simulink model "Model_Proportional"  (R2014b)
settings: Solver=ode45  StartTime=0.0  StopTime=30  RelTol=1e-6
values from neighbouring files (symbols this model uses):
  Kp = Ki    [Main.m]    (also in Q1_UsingTF.m = Kpv(i); Q2_UsingTF.m = 0; Q3_UsingTF.m; RunSimModel.m = 0)
settings Model: Creator=Eduardo  LastModifiedBy=Eduardo

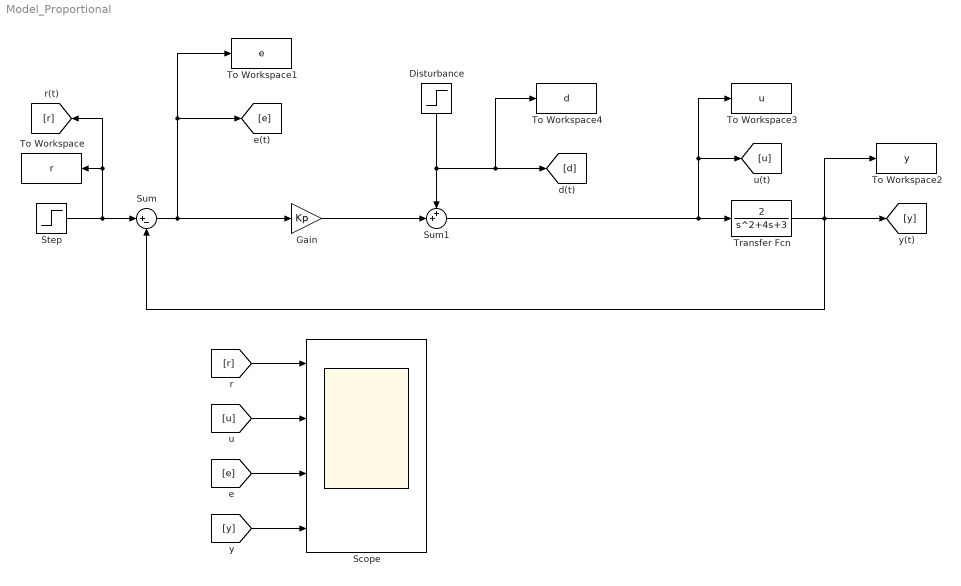
== system Model_Proportional ==
  Disturbance : Step  Time=0  After=0  SampleTime=0
  Gain : Gain  Gain=Kp
  Scope : Scope  NumInputPorts=4
      settings: YMin=-5~-5~-5~-5  YMax=5~5~5~5
  Step : Step  SampleTime=0
  Sum : Sum  Inputs=|+-
  Sum1 : Sum  Inputs=++|
  To Workspace : ToWorkspace  VariableName=r  SaveFormat=Timeseries  SampleTime=-1
  To Workspace1 : ToWorkspace  VariableName=e  SaveFormat=Timeseries  SampleTime=-1
  To Workspace2 : ToWorkspace  VariableName=y  SaveFormat=Timeseries  SampleTime=-1
  To Workspace3 : ToWorkspace  VariableName=u  SaveFormat=Timeseries  SampleTime=-1
  To Workspace4 : ToWorkspace  VariableName=d  SaveFormat=Timeseries  SampleTime=-1
  Transfer Fcn : TransferFcn  Numerator=[2]  Denominator=[1 4 3]
  wires:
  Transfer Fcn/1 -> To Workspace2/1, [y], Sum/2
  Sum/1 -> To Workspace1/1, [e], Gain/1
  [r] -> Scope/1
  [u] -> Scope/2
  [e] -> Scope/3
  [y] -> Scope/4
  Step/1 -> To Workspace/1, [r], Sum/1
  Gain/1 -> Sum1/2
  Sum1/1 -> [u], To Workspace3/1, Transfer Fcn/1
  Disturbance/1 -> To Workspace4/1, [d], Sum1/1
